simulink model "mech_airbag_vr"  (Simulink 6.0)
settings: Solver=ode45  StartTime=0.0  StopTime=3.5  RelTol=1e-6  AbsTol=1e-6
libraries: mblibv1 x38, vrlib x7, simulink x3, simulink_extras x2
settings Model: Creator=jacekk  LastModifiedBy=batserve  ExtModeAutoUpdateStatusClock=off
settings DataIOCC: SaveOutput=off  SaveTime=off  SignalLoggingName=logsOut
settings OptimizationCC: BooleanDataType=off
settings DebuggingCC: CheckExecutionContextPreStartOutputMsg=on  CheckExecutionContextRuntimeOutputMsg=on  SolverPrmCheckMsg=none
settings HardwareCC: TargetUnknown=on

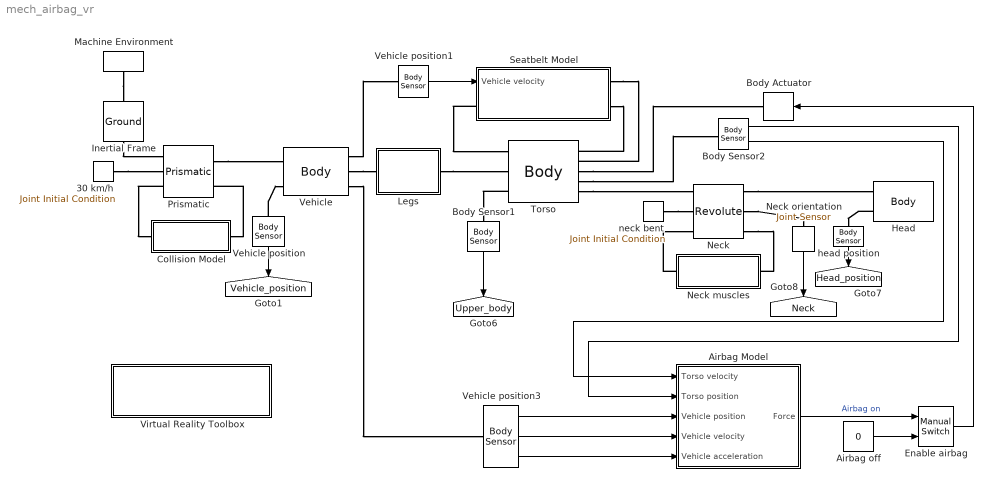
== system mech_airbag_vr ==
  30 km/h : mblibv1/Sensors &  Actuators/Joint Initial Condition  Opaque=on  PhysicalDomain=Mechanical  DialogClass=InitialConditionBlock  Primitive=P1  CoordPosition=0  Velocity=30/3.6  AngleUnits=deg  ArcVelocityUnits=deg/s  CoordPositionUnits=m  VelocityUnits=m/s  InitialConditions=P1$true$0$m$deg$30/3.6$m/s$deg/s#P2$false$0$m$rad$0$m/s$rad/s#P3$false$0$m$rad$0$m/s$rad/s#R1$false$0$m$rad$0$m/s$rad/s#R2$false$0$m$rad$0$m/s$rad/s#R3$false$0$m$rad$0$m/s$rad/s#S$false$0$m$rad$0$m/s$rad/s
  Airbag Model : Subsystem
  Airbag off : Constant  Value=0
  Body Actuator : mblibv1/Sensors &  Actuators/Body Actuator  Orientation=left  Opaque=on  PhysicalDomain=Mechanical  PortType=blob  ActuationStyle=Force  AngleUnits=deg  ArcVelocityUnits=deg/s  ArcAccelerationUnits=deg/s^2  CoordPositionUnits=m  VelocityUnits=m/s  AccelerationUnits=m/s^2  ForceUnits=N  TorqueUnits=N-m  ActiveIO=on  Width=3  DialogClass=MechanicalActuatorBlock  ReferenceFrame=Absolute (World)  Angle=off  CoordPosition=on  Force=on  Torque=off
  Body Sensor1 : mblibv1/Sensors &  Actuators/Body Sensor  Orientation=down  Opaque=on  PhysicalDomain=Mechanical  PortType=blob  Muxed=on  Pose=off  Angle=on  AngleUnits=deg  ArcVelocity=off  ArcVelocityUnits=deg/s  ArcAcceleration=off  ArcAccelerationUnits=deg/s^2  CoordPosition=on  CoordPositionUnits=cm  Velocity=off  VelocityUnits=m/s  Acceleration=off  AccelerationUnits=m/s^2  Quaternion=on  QuaternionDT=off  QuaternionDDT=off  QuaternionUnits=off  OutputVector=[ 3 ]  ActiveIO=on  Width=3  DialogClass=MechanicalSensorBlock  ReferenceFrame=Absolute (World)
  Body Sensor2 : mblibv1/Sensors &  Actuators/Body Sensor  Opaque=on  PhysicalDomain=Mechanical  PortType=blob  Muxed=off  Pose=off  Angle=on  AngleUnits=deg  ArcVelocity=off  ArcVelocityUnits=deg/s  ArcAcceleration=off  ArcAccelerationUnits=deg/s^2  CoordPosition=on  CoordPositionUnits=m  Velocity=on  VelocityUnits=m/s  Acceleration=off  AccelerationUnits=m/s^2  Quaternion=on  QuaternionDT=off  QuaternionDDT=off  QuaternionUnits=off  OutputVector=[ 3 3 ]  ActiveIO=on  Width=6  DialogClass=MechanicalSensorBlock  ReferenceFrame=Absolute (World)
  Collision Model : Subsystem
  Enable airbag : simulink/Signal Routing/Manual Switch  sw=1  action=0
  Head : mblibv1/Bodies/Body  PhysicalDomain=mechanical  SubClassName=Unknown  LeftPortType=workingframe  RightPortType=workingframe  LConnTagsString=CS1|CG  DialogClass=MechanicalBodyBlock  Mass=10  MassUnits=kg  InertiaUnits=kg*m^2  Inertia=zeros(3,3)  Shape=Cylinder  ShapeDims=[1 1]  ShapeUnits=m  ShapeUse=false  Density=1  DensityUnits=kg/m^3  DensityUse=false  CG=Left$CG$[0 15 0]$CS1$CS1$cm$[0 0 0]$Euler X-Y-Z$deg$WORLD$true  WorkingFrames=Left$CS1$[0 0 0]$ADJOINING$ADJOINING$cm$[0 0 0]$Euler X-Y-Z$deg$WORLD$true
  Inertial Frame : mblibv1/Bodies/Ground  Orientation=down  Opaque=on  LeftPortType=env  RightPortType=workingframe  PhysicalDomain=Mechanical  DialogClass=GroundBlock  CoordPosition=[0 0 0]  CoordPositionUnits=m  StateVectorMgrId=-1  MachineId=[0 0]  ShowEnvPort=on
  Legs : Subsystem
  Machine Environment : mblibv1/Bodies/Machine Environment  Tag=Factory ground  Orientation=down  DialogController=MECH.DialogSource  Opaque=on  PortType=env  PhysicalDomain=Mechanical  DialogTemplateClass=MECH.MachineEnvironment  SyncWhenCopied=off  Gravity=[0 0 0]  GravityUnits=m/s^2  GravityAsSignal=off  Dimensionality=3D Only  AnalysisType=Forward dynamics  LinearAssemblyTolerance=1e-3  LinearAssemblyToleranceUnits=m  AngularAssemblyTolerance=1e-3  AngularAssemblyToleranceUnits=rad  ConstraintSolverType=Stabilizing  ConstraintRelTolerance=1e-4  ConstraintAbsTolerance=1e-4  UseRobustSingularityHandling=off  StatePerturbationType=Adaptive  PerturbationSize=1e-3  VisualizeMachine=on
  Neck : mblibv1/Joints/Revolute  PhysicalDomain=mechanical  SubClassName=Unknown  LeftPortType=blob  RightPortType=blob  LConnTagsString=__newl0|SA1|SA2  RConnTagsString=__newr0|SA1|SA2  NumSAPorts=4  CutJoint=off  MarkAsCut=off  Primitives=revolute  PrimitiveProps=R1$Base$[0 0 1]$revolute  DialogClass=JointBlock
  Neck orientation : mblibv1/Sensors &  Actuators/Joint Sensor  Orientation=down  Opaque=on  PhysicalDomain=Mechanical  PortType=blob  Muxed=on  Pose=off  Angle=on  AngleUnits=rad  ArcVelocity=off  ArcVelocityUnits=deg/s  ArcAcceleration=off  ArcAccelerationUnits=deg/s^2  CoordPosition=on  CoordPositionUnits=m  Velocity=off  VelocityUnits=m/s  Acceleration=off  AccelerationUnits=m/s^2  Quaternion=on  QuaternionDT=off  QuaternionDDT=off  QuaternionUnits=off  OutputVector=[ 1 ]  ActiveIO=on  Width=1  DialogClass=MechanicalSensorBlock  Primitive=R1  Force=off  ForceUnits=N  Torque=off  TorqueUnits=N-m  ReferenceFrame=Absolute (INERTIAL)  ReactionSensedSide=Base  ReactionReferenceFrame=Absolute (World)  ReactionForce=off  ReactionForceUnits=N  ReactionMoment=off  ReactionMomentUnits=N-m
  Neck muscles : Subsystem  Orientation=left
  Prismatic : mblibv1/Joints/Prismatic  PhysicalDomain=mechanical  SubClassName=Unknown  LeftPortType=blob  RightPortType=blob  LConnTagsString=__newl0|SA1|SA2  RConnTagsString=__newr0|SA1  NumSAPorts=3  CutJoint=off  MarkAsCut=off  Primitives=prismatic  PrimitiveProps=P1$WORLD$[1 0 0]$prismatic  DialogClass=JointBlock
  Seatbelt Model : Subsystem
  Torso : mblibv1/Bodies/Body  PhysicalDomain=mechanical  SubClassName=Unknown  LeftPortType=workingframe  RightPortType=workingframe  LConnTagsString=CS4|CS1|CG  RConnTagsString=CS6|CS5|CS8|CS3|CS2  DialogClass=MechanicalBodyBlock  Mass=30  MassUnits=kg  InertiaUnits=kg*m^2  Inertia=zeros(3,3)  Shape=Cylinder  ShapeDims=[1 1]  ShapeUnits=m  ShapeUse=false  Density=1  DensityUnits=kg/m^3  DensityUse=false  CG=Left$CG$[0 117.5 0]$CS1$CS1$cm$[0 0 0]$Euler X-Y-Z$deg$WORLD$true  WorkingFrames=Right$CS6$[0 180 0]$CS1$CS1$cm$[0 0 0]$Euler X-Y-Z$deg$WORLD$true#Right$CS5$[0 0 0]$CS1$CS1$cm$[0 0 0]$Euler X-Y-Z$deg$WORLD$true#Left$CS4$[0 0 0]$CS1$CS1$cm$[0 0 0]$Euler X-Y-Z$deg$WORLD$true#Left$CS1$[0 0 0]$ADJOINING$ADJOINING$cm$[0 0 0]$Euler X-Y-Z$deg$WORLD$true#Right$CS8$[0 237 0]$CS1$CS1$cm$[0 0 0]$Euler X-Y-Z$deg$WORLD$true#Right$CS3$[0 237 0]$CS1$CS1$cm$[0 0 0]$Euler X-Y-Z$deg$WORLD$true#Right$CS2$[0 237 0]$CS1$CS1$cm$[0 0 0]$Euler X-Y-Z$deg$CS1$true
  Vehicle : mblibv1/Bodies/Body  PhysicalDomain=mechanical  SubClassName=Unknown  LeftPortType=workingframe  RightPortType=workingframe  LConnTagsString=CS1|CG  RConnTagsString=CS4|CS2|CS3  DialogClass=MechanicalBodyBlock  Mass=2000  MassUnits=kg  InertiaUnits=kg*m^2  Inertia=zeros(3,3)  Shape=Cylinder  ShapeDims=[1 1]  ShapeUnits=m  ShapeUse=false  Density=1  DensityUnits=kg/m^3  DensityUse=false  CG=Left$CG$[0 0 0]$WORLD$WORLD$cm$[0 0 0]$Euler X-Y-Z$deg$WORLD$true  WorkingFrames=Right$CS4$[0 0 0]$CG$CG$cm$[0 0 0]$Euler X-Y-Z$deg$WORLD$true#Left$CS1$[0 0 0]$CG$CG$cm$[0 0 0]$Euler X-Y-Z$deg$WORLD$true#Right$CS2$[10.75 -152 0]$CG$CG$cm$[0 0 0]$Euler X-Y-Z$deg$WORLD$true#Right$CS3$[0 0 0]$CG$CG$cm$[0 0 0]$Euler X-Y-Z$deg$WORLD$true
  Vehicle position : mblibv1/Sensors &  Actuators/Body Sensor  Orientation=down  Opaque=on  PhysicalDomain=Mechanical  PortType=blob  Muxed=off  Pose=off  Angle=on  AngleUnits=deg  ArcVelocity=off  ArcVelocityUnits=deg/s  ArcAcceleration=off  ArcAccelerationUnits=deg/s^2  CoordPosition=on  CoordPositionUnits=cm  Velocity=off  VelocityUnits=m/s  Acceleration=off  AccelerationUnits=m/s^2  Quaternion=on  QuaternionDT=off  QuaternionDDT=off  QuaternionUnits=off  OutputVector=[ 3 ]  ActiveIO=on  Width=3  DialogClass=MechanicalSensorBlock  ReferenceFrame=Absolute (World)
  Vehicle position1 : mblibv1/Sensors &  Actuators/Body Sensor  Opaque=on  PhysicalDomain=Mechanical  PortType=blob  Muxed=off  Pose=off  Angle=on  AngleUnits=deg  ArcVelocity=off  ArcVelocityUnits=deg/s  ArcAcceleration=off  ArcAccelerationUnits=deg/s^2  CoordPosition=off  CoordPositionUnits=cm  Velocity=on  VelocityUnits=m/s  Acceleration=off  AccelerationUnits=m/s^2  Quaternion=on  QuaternionDT=off  QuaternionDDT=off  QuaternionUnits=off  OutputVector=[ 3 ]  ActiveIO=on  Width=3  DialogClass=MechanicalSensorBlock  ReferenceFrame=Absolute (World)
  Vehicle position3 : mblibv1/Sensors &  Actuators/Body Sensor  Opaque=on  PhysicalDomain=Mechanical  PortType=blob  Muxed=off  Pose=off  Angle=on  AngleUnits=deg  ArcVelocity=off  ArcVelocityUnits=deg/s  ArcAcceleration=off  ArcAccelerationUnits=deg/s^2  CoordPosition=on  CoordPositionUnits=m  Velocity=on  VelocityUnits=m/s  Acceleration=on  AccelerationUnits=m/s^2  Quaternion=on  QuaternionDT=off  QuaternionDDT=off  QuaternionUnits=off  OutputVector=[ 3 3 3 ]  ActiveIO=on  Width=9  DialogClass=MechanicalSensorBlock  ReferenceFrame=Absolute (World)
  Virtual Reality Toolbox : Subsystem
      settings: OpenFcn=open_system([gcb '/VR Sink1']);
      mask Display: disp(sprintf('Double-click to view scene'))
  head position : mblibv1/Sensors &  Actuators/Body Sensor  Orientation=down  Opaque=on  PhysicalDomain=Mechanical  PortType=blob  Muxed=on  Pose=off  Angle=on  AngleUnits=deg  ArcVelocity=off  ArcVelocityUnits=deg/s  ArcAcceleration=off  ArcAccelerationUnits=deg/s^2  CoordPosition=on  CoordPositionUnits=cm  Velocity=off  VelocityUnits=m/s  Acceleration=off  AccelerationUnits=m/s^2  Quaternion=on  QuaternionDT=off  QuaternionDDT=off  QuaternionUnits=off  OutputVector=[ 3 ]  ActiveIO=on  Width=3  DialogClass=MechanicalSensorBlock  ReferenceFrame=Absolute (World)
  neck bent : mblibv1/Sensors &  Actuators/Joint Initial Condition  Opaque=on  PhysicalDomain=Mechanical  DialogClass=InitialConditionBlock  Primitive=R1  CoordPosition=-0.2  Velocity=0  AngleUnits=rad  ArcVelocityUnits=deg/s  CoordPositionUnits=m  VelocityUnits=m/s  InitialConditions=P1$false$0$m$rad$0$m/s$rad/s#P2$false$0$m$rad$0$m/s$rad/s#P3$false$0$m$rad$0$m/s$rad/s#R1$true$-0.2$m$rad$0$m/s$deg/s#R2$false$0$m$rad$0$m/s$rad/s#R3$false$0$m$rad$0$m/s$rad/s#S$false$0$m$rad$0$m/s$rad/s
  tag scope: Head_position=global, Neck=global, Upper_body=global, Vehicle_position=global
  wires:
  Vehicle position/1 -> [Vehicle_position]
  Body Sensor1/1 -> [Upper_body]
  head position/1 -> [Head_position]
  Neck orientation/1 -> [Neck]
  Vehicle position1/1 -> Seatbelt Model/1(Vehicle velocity)
  Vehicle position3/1 -> Airbag Model/3(Vehicle position)
  Vehicle position3/2 -> Airbag Model/4(Vehicle velocity)
  Vehicle position3/3 -> Airbag Model/5(Vehicle acceleration)
  Body Sensor2/2 -> Airbag Model/1(Torso velocity)
  Body Sensor2/1 -> Airbag Model/2(Torso position)
  Airbag Model/1(Force) -> Enable airbag/1  "Airbag on"
  Airbag off/1 -> Enable airbag/2
  Enable airbag/1 -> Body Actuator/1
  connections:
  Torso/RConn5 -- Neck/LConn1
  Neck/RConn1 -- Head/LConn1
  Inertial Frame/RConn1 -- Prismatic/LConn1
  Prismatic/RConn1 -- Vehicle/LConn1
  30 km/h/RConn1 -- Prismatic/LConn2
  Collision Model/RConn1 -- Prismatic/RConn2
  Torso/LConn3 -- Body Sensor1/LConn1
  Head/LConn2 -- head position/LConn1
  Vehicle position/LConn1 -- Vehicle/LConn2
  Neck/RConn3 -- Neck muscles/LConn1
  Neck muscles/RConn1 -- Neck/LConn3
  neck bent/RConn1 -- Neck/LConn2
  Neck/RConn2 -- Neck orientation/LConn1
  Seatbelt Model/RConn1 -- Torso/RConn2
  Vehicle/RConn1 -- Vehicle position1/LConn1
  Seatbelt Model/RConn2 -- Torso/RConn1
  Vehicle/RConn3 -- Vehicle position3/LConn1
  Prismatic/LConn3 -- Collision Model/LConn1
  Vehicle/RConn2 -- Legs/LConn1
  Seatbelt Model/LConn1 -- Torso/LConn1
  Torso/RConn4 -- Body Sensor2/LConn1
  Torso/RConn3 -- Body Actuator/RConn1
  Legs/RConn1 -- Torso/LConn2
  Machine Environment/RConn1 -- Inertial Frame/LConn1

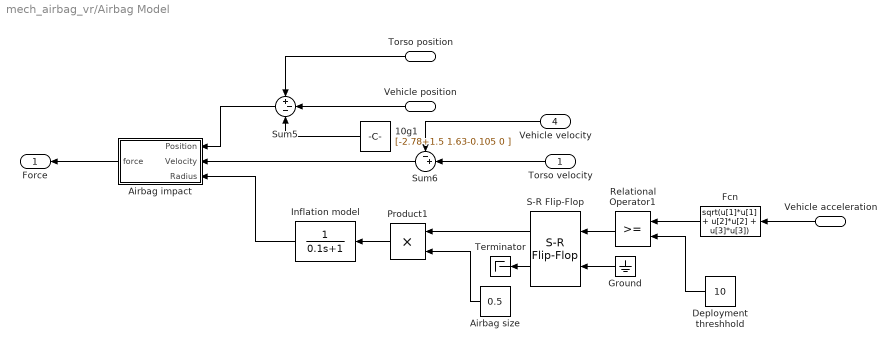
== system mech_airbag_vr/Airbag Model ==
  Torso velocity : Inport  Orientation=left  Port=1  LatchInput=off
  Torso position : Inport  Orientation=left  Port=2  LatchInput=off
  Vehicle position : Inport  Orientation=left  Port=3  LatchInput=off
  Vehicle velocity : Inport  Orientation=left  Port=4  LatchInput=off
  Vehicle acceleration : Inport  Orientation=left  Port=5  LatchInput=off
  10g1 : Constant  Orientation=left  Value=[-2.78+1.5 1.63-0.105 0 ]
  Airbag size : Constant  Orientation=left  Value=0.5
  Airbag impact : Subsystem  Orientation=left
  Deployment threshhold : Constant  Orientation=left  Value=10
  Fcn : Fcn  Orientation=left  Expr=sqrt(u[1]*u[1] + u[2]*u[2] + u[3]*u[3])
  Ground : Ground  Orientation=left
  Inflation model : TransferFcn  Orientation=left  Denominator=[0.1 1]
  Product1 : Product  Orientation=left  SaturateOnIntegerOverflow=on  InputSameDT=on
  Relational Operator1 : RelationalOperator  Orientation=left  ZeroCross=off  InputSameDT=on
  S-R Flip-Flop : simulink_extras/Flip Flops/S-R Flip-Flop  Orientation=left  initial_condition=0
  Sum5 : Sum  Orientation=left  Inputs=+--  SaturateOnIntegerOverflow=on  InputSameDT=on
  Sum6 : Sum  Orientation=left  Inputs=-+|  SaturateOnIntegerOverflow=on  InputSameDT=on
  Terminator : Terminator
  Force : Outport  Orientation=left
  wires:
  10g1/1 -> Sum5/3
  Sum6/1 -> Airbag impact/2(Velocity)
  S-R Flip-Flop/1 -> Product1/1
  Product1/1 -> Inflation model/1
  Vehicle position/1 -> Sum5/2
  Airbag impact/1(force) -> Force/1
  Relational Operator1/1 -> S-R Flip-Flop/1
  Fcn/1 -> Relational Operator1/1
  Vehicle acceleration/1 -> Fcn/1
  Torso velocity/1 -> Sum6/2
  Sum5/1 -> Airbag impact/1(Position)
  Torso position/1 -> Sum5/1
  Inflation model/1 -> Airbag impact/3(Radius)
  Airbag size/1 -> Product1/2
  Deployment threshhold/1 -> Relational Operator1/2
  Vehicle velocity/1 -> Sum6/1
  S-R Flip-Flop/2 -> Terminator/1
  Ground/1 -> S-R Flip-Flop/2

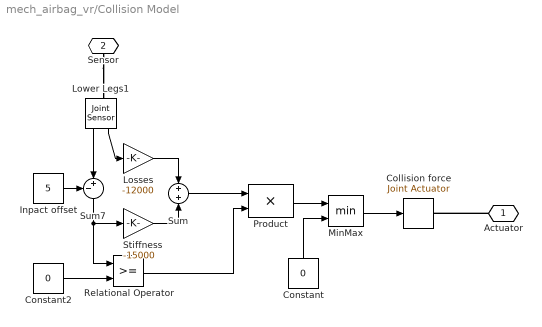
== system mech_airbag_vr/Collision Model ==
  Collision force : mblibv1/Sensors &  Actuators/Joint Actuator  Opaque=on  PhysicalDomain=Mechanical  PortType=blob  ActuationStyle=Force  AngleUnits=deg  ArcVelocityUnits=deg/s  ArcAccelerationUnits=deg/s^2  CoordPositionUnits=m  VelocityUnits=m/s  AccelerationUnits=m/s^2  ForceUnits=N  TorqueUnits=N-m  ActiveIO=on  Width=1  DialogClass=MechanicalActuatorBlock  Primitive=P1  ReferenceFrame=Absolute (INERTIAL)
  Constant : Constant  Orientation=up  Value=0
  Constant2 : Constant  Value=0
  Inpact offset : Constant  Value=5
  Losses : Gain  Gain=-12000  SaturateOnIntegerOverflow=on
  Lower Legs1 : mblibv1/Sensors &  Actuators/Joint Sensor  Orientation=down  Opaque=on  PhysicalDomain=Mechanical  PortType=blob  Muxed=off  Pose=off  Angle=on  AngleUnits=rad  ArcVelocity=off  ArcVelocityUnits=deg/s  ArcAcceleration=off  ArcAccelerationUnits=deg/s^2  CoordPosition=on  CoordPositionUnits=m  Velocity=on  VelocityUnits=m/s  Acceleration=off  AccelerationUnits=m/s^2  Quaternion=on  QuaternionDT=off  QuaternionDDT=off  QuaternionUnits=off  OutputVector=[ 1 1 ]  ActiveIO=on  Width=2  DialogClass=MechanicalSensorBlock  Primitive=P1  Force=off  ForceUnits=N  Torque=off  TorqueUnits=N-m  ReferenceFrame=Absolute (INERTIAL)  ReactionSensedSide=Base  ReactionReferenceFrame=Absolute (World)  ReactionForce=off  ReactionForceUnits=N  ReactionMoment=off  ReactionMomentUnits=N-m
  MinMax : MinMax  Inputs=2  ZeroCross=off  SaturateOnIntegerOverflow=on  InputSameDT=on
  Product : Product  SaturateOnIntegerOverflow=on  InputSameDT=on
  Relational Operator : RelationalOperator  ZeroCross=off  InputSameDT=on
  Stiffness : Gain  Gain=-15000  SaturateOnIntegerOverflow=on
  Sum : Sum  SaturateOnIntegerOverflow=on  InputSameDT=on
  Sum7 : Sum  Orientation=down  Inputs=-+|  SaturateOnIntegerOverflow=on  InputSameDT=on
  Actuator : PMIOPort  Orientation=left  Port=1  Side=Right
  Sensor : PMIOPort  Orientation=down  Port=2  Side=Left
  wires:
  MinMax/1 -> Collision force/1
  Lower Legs1/2 -> Losses/1
  Stiffness/1 -> Sum/2
  Relational Operator/1 -> Product/2
  Sum/1 -> Product/1
  Lower Legs1/1 -> Sum7/2
  Inpact offset/1 -> Sum7/1
  Sum7/1 -> Relational Operator/1, Stiffness/1
  Constant2/1 -> Relational Operator/2
  Product/1 -> MinMax/1
  Losses/1 -> Sum/1
  Constant/1 -> MinMax/2
  connections:
  Actuator/RConn1 -- Collision force/RConn1
  Sensor/RConn1 -- Lower Legs1/LConn1

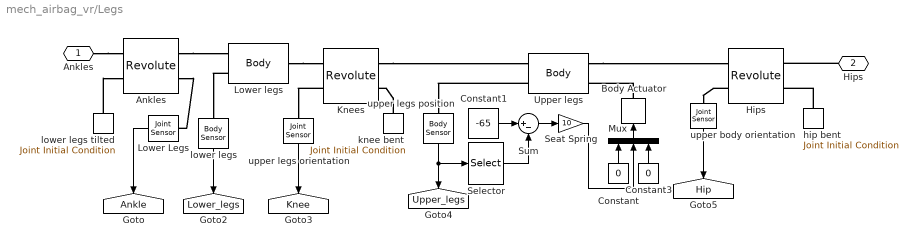
== system mech_airbag_vr/Legs ==
  Ankles : mblibv1/Joints/Revolute  PhysicalDomain=mechanical  SubClassName=Unknown  LeftPortType=blob  RightPortType=blob  LConnTagsString=__newl0|SA1  RConnTagsString=__newr0|SA1  NumSAPorts=2  CutJoint=off  MarkAsCut=off  Primitives=revolute  PrimitiveProps=R1$Base$[0 0 1]$revolute  DialogClass=JointBlock
  Body Actuator : mblibv1/Sensors &  Actuators/Body Actuator  Orientation=up  Opaque=on  PhysicalDomain=Mechanical  PortType=blob  ActuationStyle=Force  AngleUnits=deg  ArcVelocityUnits=deg/s  ArcAccelerationUnits=deg/s^2  CoordPositionUnits=m  VelocityUnits=m/s  AccelerationUnits=m/s^2  ForceUnits=N  TorqueUnits=N-m  ActiveIO=on  Width=3  DialogClass=MechanicalActuatorBlock  ReferenceFrame=Absolute (World)  Angle=off  CoordPosition=on  Force=on  Torque=off
  Constant : Constant  Orientation=up  Value=0
  Constant1 : Constant  Value=-65
  Constant3 : Constant  Orientation=up  Value=0
  Hips : mblibv1/Joints/Revolute  PhysicalDomain=mechanical  SubClassName=Unknown  LeftPortType=blob  RightPortType=blob  LConnTagsString=__newl0|SA1  RConnTagsString=__newr0|SA1  NumSAPorts=2  CutJoint=off  MarkAsCut=off  Primitives=revolute  PrimitiveProps=R1$Base$[0 0 1]$revolute  DialogClass=JointBlock
  Knees : mblibv1/Joints/Revolute  PhysicalDomain=mechanical  SubClassName=Unknown  LeftPortType=blob  RightPortType=blob  LConnTagsString=__newl0|SA1  RConnTagsString=__newr0|SA1  NumSAPorts=2  CutJoint=off  MarkAsCut=off  Primitives=revolute  PrimitiveProps=R1$Base$[0 0 1]$revolute  DialogClass=JointBlock
  Lower Legs : mblibv1/Sensors &  Actuators/Joint Sensor  Orientation=left  Opaque=on  PhysicalDomain=Mechanical  PortType=blob  Muxed=on  Pose=off  Angle=on  AngleUnits=rad  ArcVelocity=off  ArcVelocityUnits=deg/s  ArcAcceleration=off  ArcAccelerationUnits=deg/s^2  CoordPosition=on  CoordPositionUnits=m  Velocity=off  VelocityUnits=m/s  Acceleration=off  AccelerationUnits=m/s^2  Quaternion=on  QuaternionDT=off  QuaternionDDT=off  QuaternionUnits=off  OutputVector=[ 1 ]  ActiveIO=on  Width=1  DialogClass=MechanicalSensorBlock  Primitive=R1  Force=off  ForceUnits=N  Torque=off  TorqueUnits=N-m  ReferenceFrame=Absolute (INERTIAL)  ReactionSensedSide=Base  ReactionReferenceFrame=Absolute (World)  ReactionForce=off  ReactionForceUnits=N  ReactionMoment=off  ReactionMomentUnits=N-m
  Lower legs : mblibv1/Bodies/Body  PhysicalDomain=mechanical  SubClassName=Unknown  LeftPortType=workingframe  RightPortType=workingframe  LConnTagsString=CS1|CG  RConnTagsString=CS2  DialogClass=MechanicalBodyBlock  Mass=5  MassUnits=kg  InertiaUnits=kg*m^2  Inertia=zeros(3,3)  Shape=Cylinder  ShapeDims=[1 1]  ShapeUnits=m  ShapeUse=false  Density=1  DensityUnits=kg/m^3  DensityUse=false  CG=Left$CG$[0 60 0]$CS1$CS1$cm$[0 0 0]$Euler X-Y-Z$deg$CS1$true  WorkingFrames=Left$CS1$[0 0 0]$ADJOINING$ADJOINING$cm$[0 0 0]$Euler X-Y-Z$deg$ADJOINING$true#Right$CS2$[0 120 0]$CS1$CS1$cm$[0 0 0]$Euler X-Y-Z$deg$CS1$true
  Mux : Mux  Orientation=up  Inputs=3
  Seat Spring : Gain  Gain=10  SaturateOnIntegerOverflow=on
  Selector : Selector  Elements=2  InputPortWidth=3
  Sum : Sum  Inputs=|+-  SaturateOnIntegerOverflow=on  InputSameDT=on
  Upper legs : mblibv1/Bodies/Body  PhysicalDomain=mechanical  SubClassName=Unknown  LeftPortType=workingframe  RightPortType=workingframe  LConnTagsString=CS1|CG  RConnTagsString=CS2|CS3  DialogClass=MechanicalBodyBlock  Mass=15  MassUnits=kg  InertiaUnits=kg*m^2  Inertia=zeros(3,3)  Shape=Cylinder  ShapeDims=[1 1]  ShapeUnits=m  ShapeUse=false  Density=1  DensityUnits=kg/m^3  DensityUse=false  CG=Left$CG$[0 94 0]$CS1$CS1$cm$[0 0 0]$Euler X-Y-Z$deg$CS1$true  WorkingFrames=Left$CS1$[0 0 0]$ADJOINING$ADJOINING$cm$[0 0 0]$Euler X-Y-Z$deg$ADJOINING$true#Right$CS2$[0 188 0]$CS1$CS1$cm$[0 0 0]$Euler X-Y-Z$deg$CS1$true#Right$CS3$[0 188 0]$CS1$CS1$cm$[0 0 0]$Euler X-Y-Z$deg$CS1$true
  hip bent : mblibv1/Sensors &  Actuators/Joint Initial Condition  Orientation=up  Opaque=on  PhysicalDomain=Mechanical  DialogClass=InitialConditionBlock  Primitive=R1  CoordPosition=-1.57  Velocity=0  AngleUnits=rad  ArcVelocityUnits=deg/s  CoordPositionUnits=m  VelocityUnits=m/s  InitialConditions=P1$false$0$m$rad$0$m/s$rad/s#P2$false$0$m$rad$0$m/s$rad/s#P3$false$0$m$rad$0$m/s$rad/s#R1$true$-1.57$m$rad$0$m/s$deg/s#R2$false$0$m$rad$0$m/s$rad/s#R3$false$0$m$rad$0$m/s$rad/s#S$false$0$m$rad$0$m/s$rad/s
  knee bent : mblibv1/Sensors &  Actuators/Joint Initial Condition  Orientation=up  Opaque=on  PhysicalDomain=Mechanical  DialogClass=InitialConditionBlock  Primitive=R1  CoordPosition=1.27  Velocity=0  AngleUnits=rad  ArcVelocityUnits=deg/s  CoordPositionUnits=m  VelocityUnits=m/s  InitialConditions=P1$false$0$m$rad$0$m/s$rad/s#P2$false$0$m$rad$0$m/s$rad/s#P3$false$0$m$rad$0$m/s$rad/s#R1$true$1.27$m$rad$0$m/s$deg/s#R2$false$0$m$rad$0$m/s$rad/s#R3$false$0$m$rad$0$m/s$rad/s#S$false$0$m$rad$0$m/s$rad/s
  "lower legs " : mblibv1/Sensors &  Actuators/Body Sensor  Orientation=down  Opaque=on  PhysicalDomain=Mechanical  PortType=blob  Muxed=on  Pose=off  Angle=on  AngleUnits=deg  ArcVelocity=off  ArcVelocityUnits=deg/s  ArcAcceleration=off  ArcAccelerationUnits=deg/s^2  CoordPosition=on  CoordPositionUnits=cm  Velocity=off  VelocityUnits=m/s  Acceleration=off  AccelerationUnits=m/s^2  Quaternion=on  QuaternionDT=off  QuaternionDDT=off  QuaternionUnits=off  OutputVector=[ 3 ]  ActiveIO=on  Width=3  DialogClass=MechanicalSensorBlock  ReferenceFrame=Absolute (World)
  lower legs tilted : mblibv1/Sensors &  Actuators/Joint Initial Condition  Orientation=up  Opaque=on  PhysicalDomain=Mechanical  DialogClass=InitialConditionBlock  Primitive=R1  CoordPosition=0.5  Velocity=0  AngleUnits=rad  ArcVelocityUnits=deg/s  CoordPositionUnits=m  VelocityUnits=m/s  InitialConditions=P1$false$0$m$rad$0$m/s$rad/s#P2$false$0$m$rad$0$m/s$rad/s#P3$false$0$m$rad$0$m/s$rad/s#R1$true$0.5$m$rad$0$m/s$deg/s#R2$false$0$m$rad$0$m/s$rad/s#R3$false$0$m$rad$0$m/s$rad/s#S$false$0$m$rad$0$m/s$rad/s
  upper body orientation : mblibv1/Sensors &  Actuators/Joint Sensor  Orientation=down  Opaque=on  PhysicalDomain=Mechanical  PortType=blob  Muxed=on  Pose=off  Angle=on  AngleUnits=rad  ArcVelocity=off  ArcVelocityUnits=deg/s  ArcAcceleration=off  ArcAccelerationUnits=deg/s^2  CoordPosition=on  CoordPositionUnits=m  Velocity=off  VelocityUnits=m/s  Acceleration=off  AccelerationUnits=m/s^2  Quaternion=on  QuaternionDT=off  QuaternionDDT=off  QuaternionUnits=off  OutputVector=[ 1 ]  ActiveIO=on  Width=1  DialogClass=MechanicalSensorBlock  Primitive=R1  Force=off  ForceUnits=N  Torque=off  TorqueUnits=N-m  ReferenceFrame=Absolute (INERTIAL)  ReactionSensedSide=Base  ReactionReferenceFrame=Absolute (World)  ReactionForce=off  ReactionForceUnits=N  ReactionMoment=off  ReactionMomentUnits=N-m
  upper legs orientation : mblibv1/Sensors &  Actuators/Joint Sensor  Orientation=down  Opaque=on  PhysicalDomain=Mechanical  PortType=blob  Muxed=on  Pose=off  Angle=on  AngleUnits=rad  ArcVelocity=off  ArcVelocityUnits=deg/s  ArcAcceleration=off  ArcAccelerationUnits=deg/s^2  CoordPosition=on  CoordPositionUnits=m  Velocity=off  VelocityUnits=m/s  Acceleration=off  AccelerationUnits=m/s^2  Quaternion=on  QuaternionDT=off  QuaternionDDT=off  QuaternionUnits=off  OutputVector=[ 1 ]  ActiveIO=on  Width=1  DialogClass=MechanicalSensorBlock  Primitive=R1  Force=off  ForceUnits=N  Torque=off  TorqueUnits=N-m  ReferenceFrame=Absolute (INERTIAL)  ReactionSensedSide=Base  ReactionReferenceFrame=Absolute (World)  ReactionForce=off  ReactionForceUnits=N  ReactionMoment=off  ReactionMomentUnits=N-m
  upper legs position : mblibv1/Sensors &  Actuators/Body Sensor  Orientation=down  Opaque=on  PhysicalDomain=Mechanical  PortType=blob  Muxed=on  Pose=off  Angle=on  AngleUnits=deg  ArcVelocity=off  ArcVelocityUnits=deg/s  ArcAcceleration=off  ArcAccelerationUnits=deg/s^2  CoordPosition=on  CoordPositionUnits=cm  Velocity=off  VelocityUnits=m/s  Acceleration=off  AccelerationUnits=m/s^2  Quaternion=on  QuaternionDT=off  QuaternionDDT=off  QuaternionUnits=off  OutputVector=[ 3 ]  ActiveIO=on  Width=3  DialogClass=MechanicalSensorBlock  ReferenceFrame=Absolute (World)
  "Ankles  " : PMIOPort  Port=1  Side=Left
  "Hips " : PMIOPort  Orientation=left  Port=2  Side=Right
  tag scope: Ankle=global, Hip=global, Knee=global, Lower_legs=global, Upper_legs=global
  wires:
  Lower Legs/1 -> [Ankle]
  "lower legs "/1 -> [Lower_legs]
  upper legs orientation/1 -> [Knee]
  upper legs position/1 -> [Upper_legs], Selector/1
  upper body orientation/1 -> [Hip]
  Constant1/1 -> Sum/1
  Selector/1 -> Sum/2
  Sum/1 -> Seat Spring/1
  Mux/1 -> Body Actuator/1
  Constant/1 -> Mux/1
  Constant3/1 -> Mux/3
  Seat Spring/1 -> Mux/2
  connections:
  Lower legs/RConn1 -- Knees/LConn1
  Knees/RConn1 -- Upper legs/LConn1
  Upper legs/RConn1 -- Hips/LConn1
  knee bent/RConn1 -- Knees/RConn2
  hip bent/RConn1 -- Hips/RConn2
  Lower legs/LConn2 -- "lower legs "/LConn1
  Upper legs/LConn2 -- upper legs position/LConn1
  Hips/LConn2 -- upper body orientation/LConn1
  Ankles/RConn1 -- Lower legs/LConn1
  lower legs tilted/RConn1 -- Ankles/LConn2
  Ankles/RConn2 -- Lower Legs/LConn1
  Knees/LConn2 -- upper legs orientation/LConn1
  "Ankles  "/RConn1 -- Ankles/LConn1
  "Hips "/RConn1 -- Hips/RConn1
  Body Actuator/RConn1 -- Upper legs/RConn2

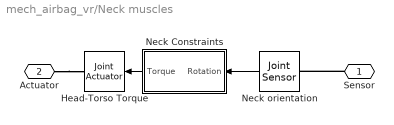
== system mech_airbag_vr/Neck muscles ==
  Head-Torso Torque : mblibv1/Sensors &  Actuators/Joint Actuator  Orientation=left  Opaque=on  PhysicalDomain=Mechanical  PortType=blob  ActuationStyle=Force  AngleUnits=deg  ArcVelocityUnits=deg/s  ArcAccelerationUnits=deg/s^2  CoordPositionUnits=m  VelocityUnits=m/s  AccelerationUnits=m/s^2  ForceUnits=N  TorqueUnits=N-m  ActiveIO=on  Width=1  DialogClass=MechanicalActuatorBlock  Primitive=R1  ReferenceFrame=Absolute (INERTIAL)
  Neck Constraints : Subsystem  Orientation=left
  Neck orientation : mblibv1/Sensors &  Actuators/Joint Sensor  Orientation=left  Opaque=on  PhysicalDomain=Mechanical  PortType=blob  Muxed=on  Pose=off  Angle=on  AngleUnits=rad  ArcVelocity=on  ArcVelocityUnits=rad/s  ArcAcceleration=off  ArcAccelerationUnits=deg/s^2  CoordPosition=on  CoordPositionUnits=m  Velocity=off  VelocityUnits=m/s  Acceleration=off  AccelerationUnits=m/s^2  Quaternion=on  QuaternionDT=off  QuaternionDDT=off  QuaternionUnits=off  OutputVector=[ 1 1 ]  ActiveIO=on  Width=2  DialogClass=MechanicalSensorBlock  Primitive=R1  Force=off  ForceUnits=N  Torque=off  TorqueUnits=N-m  ReferenceFrame=Absolute (INERTIAL)  ReactionSensedSide=Base  ReactionReferenceFrame=Absolute (World)  ReactionForce=off  ReactionForceUnits=N  ReactionMoment=off  ReactionMomentUnits=N-m
  Sensor : PMIOPort  Orientation=left  Port=1  Side=Left
  Actuator : PMIOPort  Port=2  Side=Right
  wires:
  Neck Constraints/1(Torque) -> Head-Torso Torque/1
  Neck orientation/1 -> Neck Constraints/1(Rotation)
  connections:
  Sensor/RConn1 -- Neck orientation/LConn1
  Actuator/RConn1 -- Head-Torso Torque/RConn1

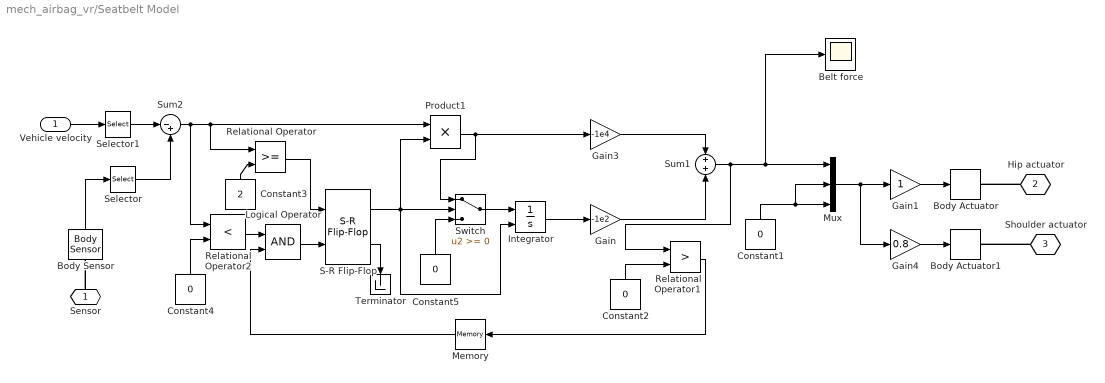
== system mech_airbag_vr/Seatbelt Model ==
  Vehicle velocity : Inport  Port=1  LatchInput=off
  Belt force : Scope
      settings: TimeRange=1  YMin=-25000  YMax=5000
  Body Actuator : mblibv1/Sensors &  Actuators/Body Actuator  Opaque=on  PhysicalDomain=Mechanical  PortType=blob  ActuationStyle=Force  AngleUnits=deg  ArcVelocityUnits=deg/s  ArcAccelerationUnits=deg/s^2  CoordPositionUnits=m  VelocityUnits=m/s  AccelerationUnits=m/s^2  ForceUnits=N  TorqueUnits=N-m  ActiveIO=on  Width=3  DialogClass=MechanicalActuatorBlock  ReferenceFrame=Local (Body CS)  Angle=off  CoordPosition=on  Force=on  Torque=off
  Body Actuator1 : mblibv1/Sensors &  Actuators/Body Actuator  Opaque=on  PhysicalDomain=Mechanical  PortType=blob  ActuationStyle=Force  AngleUnits=deg  ArcVelocityUnits=deg/s  ArcAccelerationUnits=deg/s^2  CoordPositionUnits=m  VelocityUnits=m/s  AccelerationUnits=m/s^2  ForceUnits=N  TorqueUnits=N-m  ActiveIO=on  Width=3  DialogClass=MechanicalActuatorBlock  ReferenceFrame=Absolute (World)  Angle=off  CoordPosition=on  Force=on  Torque=off
  Body Sensor : mblibv1/Sensors &  Actuators/Body Sensor  Orientation=up  Opaque=on  PhysicalDomain=Mechanical  PortType=blob  Muxed=off  Pose=off  Angle=on  AngleUnits=deg  ArcVelocity=off  ArcVelocityUnits=deg/s  ArcAcceleration=off  ArcAccelerationUnits=deg/s^2  CoordPosition=off  CoordPositionUnits=cm  Velocity=on  VelocityUnits=m/s  Acceleration=off  AccelerationUnits=m/s^2  Quaternion=on  QuaternionDT=off  QuaternionDDT=off  QuaternionUnits=off  OutputVector=[ 3 ]  ActiveIO=on  Width=3  DialogClass=MechanicalSensorBlock  ReferenceFrame=Absolute (World)
  Constant{1..2,4..5} (4 alike) : Constant  Orientation=up  Value=0
  Constant3 : Constant  Orientation=up  Value=2
  Gain : Gain  Gain=-1e2  SaturateOnIntegerOverflow=on
  Gain1 : Gain  SaturateOnIntegerOverflow=on
  Gain3 : Gain  Gain=-1e4  SaturateOnIntegerOverflow=on
  Gain4 : Gain  Gain=0.8  SaturateOnIntegerOverflow=on
  Integrator : Integrator  ExternalReset=either  AbsoluteTolerance=1e-8  ZeroCross=off
  Logical Operator : Logic
  Memory : Memory  Orientation=left
  Mux : Mux  Inputs=3
  Product1 : Product  SaturateOnIntegerOverflow=on  InputSameDT=on
  Relational Operator : RelationalOperator  ZeroCross=off  InputSameDT=on
  Relational Operator1 : RelationalOperator  Operator=>  ZeroCross=off  InputSameDT=on
  Relational Operator2 : RelationalOperator  Operator=<  ZeroCross=off  InputSameDT=on
  S-R Flip-Flop : simulink_extras/Flip Flops/S-R Flip-Flop  initial_condition=0
  Selector : Selector  InputPortWidth=3
  Selector1 : Selector  InputPortWidth=3
  Sum1 : Sum  SaturateOnIntegerOverflow=on  InputSameDT=on
  Sum2 : Sum  Inputs=|-+  SaturateOnIntegerOverflow=on  InputSameDT=on
  Switch : Switch  ZeroCross=off  InputSameDT=on
  Terminator : Terminator
      settings: Orientation=down
  Sensor : PMIOPort  Orientation=up  Port=1  Side=Left
  Hip actuator : PMIOPort  Orientation=left  Port=2  Side=Right
  Shoulder actuator : PMIOPort  Orientation=left  Port=3  Side=Right
  wires:
  Vehicle velocity/1 -> Selector1/1
  Gain1/1 -> Body Actuator/1
  Relational Operator/1 -> S-R Flip-Flop/1
  Constant3/1 -> Relational Operator/2
  Sum1/1 -> Relational Operator1/1, Mux/1, Belt force/1
  Constant1/1 -> Mux/3, Mux/2
  Constant2/1 -> Relational Operator1/2
  Body Sensor/1 -> Selector/1
  Integrator/1 -> Gain/1
  Gain/1 -> Sum1/2
  S-R Flip-Flop/1 -> Product1/2, Switch/2, Integrator/2
  Logical Operator/1 -> S-R Flip-Flop/2
  Relational Operator2/1 -> Logical Operator/1
  Relational Operator1/1 -> Memory/1
  Gain3/1 -> Sum1/1
  Mux/1 -> Gain1/1, Gain4/1
  Memory/1 -> Logical Operator/2
  Selector1/1 -> Sum2/1
  Selector/1 -> Sum2/2
  Sum2/1 -> Relational Operator2/1, Relational Operator/1, Product1/1
  Constant4/1 -> Relational Operator2/2
  Gain4/1 -> Body Actuator1/1
  Product1/1 -> Gain3/1, Switch/1
  Switch/1 -> Integrator/1
  Constant5/1 -> Switch/3
  S-R Flip-Flop/2 -> Terminator/1
  connections:
  Sensor/RConn1 -- Body Sensor/LConn1
  Hip actuator/RConn1 -- Body Actuator/RConn1
  Shoulder actuator/RConn1 -- Body Actuator1/RConn1

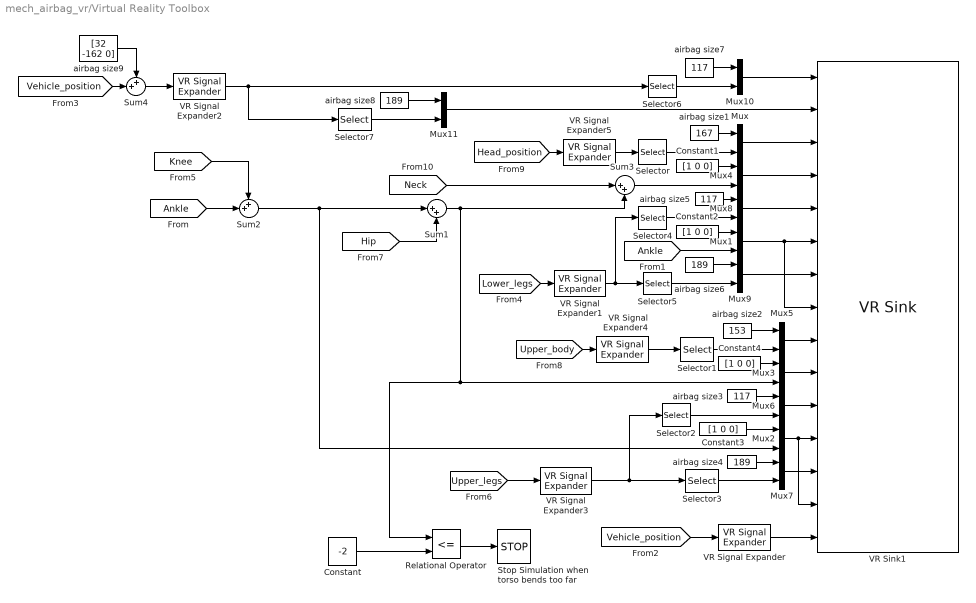
== system mech_airbag_vr/Virtual Reality Toolbox ==
  Constant : Constant  Value=-2
  Constant{1..4} (4 alike) : Constant  Value=[1 0 0]
  Mux{,1..11} (12 alike) : Mux  Inputs=2
  Relational Operator : RelationalOperator  Operator=<=  ZeroCross=off  InputSameDT=on
  Selector{,1..7} (8 alike) : Selector  Elements=[2 3]  InputPortWidth=3
  Stop Simulation when torso bends too far : Stop
  Sum1 : Sum  Inputs=|++  SaturateOnIntegerOverflow=on  InputSameDT=on
  Sum2 : Sum  Inputs=++|  SaturateOnIntegerOverflow=on  InputSameDT=on
  Sum3 : Sum  Inputs=|++  SaturateOnIntegerOverflow=on  InputSameDT=on
  Sum4 : Sum  Inputs=++|  SaturateOnIntegerOverflow=on  InputSameDT=on
  VR Signal Expander{,1..5} (6 alike) : vrlib/VR Signal Expander  outwidth=3  outidx=[2 3 1]
  VR Sink1 : vrlib/VR Sink  SampleTime=0.05  ViewEnable=on  RemoteChange=off  RemoteView=off  FieldsWritten=footL.translation#footR.translation#headCOG.translation#headROT.rotation#lowerlegL.translation#lowerlegLROT.rotation#lowerlegR.translation#lowerlegRROT.rotation#torsoCOG.translation#torsoROT.rotation#upperlegL.translation#upperlegLROT.rotation#upperlegR.translation#upperlegRROT.rotation#vehicle.translation  WorldFileName=mech_airbag_world.wrl  WorldDescription=Passenger Collision Model  AutoView=off  FigureProperties={}
  airbag size1 : Constant  Value=167
  airbag size2 : Constant  Value=153
  airbag size3 : Constant  Value=117
  airbag size4 : Constant  Value=189
  airbag size5 : Constant  Value=117
  airbag size6 : Constant  Value=189
  airbag size7 : Constant  Value=117
  airbag size8 : Constant  Value=189
  airbag size9 : Constant  Value=[32 -162 0]
  wires:
  Sum3/1 -> Mux4/2
  Mux4/1 -> VR Sink1/4
  Mux3/1 -> VR Sink1/10
  airbag size1/1 -> Mux/1
  Selector/1 -> Mux/2
  Mux/1 -> VR Sink1/3
  Selector1/1 -> Mux5/2
  airbag size3/1 -> Mux6/1
  airbag size4/1 -> Mux7/1
  airbag size6/1 -> Mux9/1
  Selector4/1 -> Mux8/2
  Selector5/1 -> Mux9/2
  Selector7/1 -> Mux11/2
  airbag size8/1 -> Mux11/1
  airbag size7/1 -> Mux10/1
  [Ankle] -> Sum2/2
  [Ankle] -> Mux1/2
  [Vehicle_position] -> VR Signal Expander/1
  [Vehicle_position] -> Sum4/2
  Sum4/1 -> VR Signal Expander2/1
  airbag size9/1 -> Sum4/1
  [Lower_legs] -> VR Signal Expander1/1
  [Hip] -> Sum1/2
  [Upper_body] -> VR Signal Expander4/1
  [Head_position] -> VR Signal Expander5/1
  [Neck] -> Sum3/1
  Selector6/1 -> Mux10/2
  VR Signal Expander2/1 -> Selector7/1, Selector6/1
  VR Signal Expander5/1 -> Selector/1
  Mux10/1 -> VR Sink1/1
  Mux11/1 -> VR Sink1/2
  Constant1/1 -> Mux4/1
  Mux8/1 -> VR Sink1/5
  airbag size5/1 -> Mux8/1
  Mux9/1 -> VR Sink1/7
  Mux1/1 -> VR Sink1/6, VR Sink1/8
  Constant2/1 -> Mux1/1
  Constant4/1 -> Mux3/1
  VR Signal Expander1/1 -> Selector5/1, Selector4/1
  Mux5/1 -> VR Sink1/9
  airbag size2/1 -> Mux5/1
  VR Signal Expander4/1 -> Selector1/1
  Constant3/1 -> Mux2/1
  Mux2/1 -> VR Sink1/12, VR Sink1/14
  [Knee] -> Sum2/1
  Sum1/1 -> Sum3/2, Relational Operator/1, Mux3/2
  Sum2/1 -> Sum1/1, Mux2/2
  Mux6/1 -> VR Sink1/11
  Selector2/1 -> Mux6/2
  Mux7/1 -> VR Sink1/13
  Selector3/1 -> Mux7/2
  VR Signal Expander/1 -> VR Sink1/15
  VR Signal Expander3/1 -> Selector3/1, Selector2/1
  [Upper_legs] -> VR Signal Expander3/1
  Constant/1 -> Relational Operator/2
  Relational Operator/1 -> Stop Simulation when torso bends too far/1

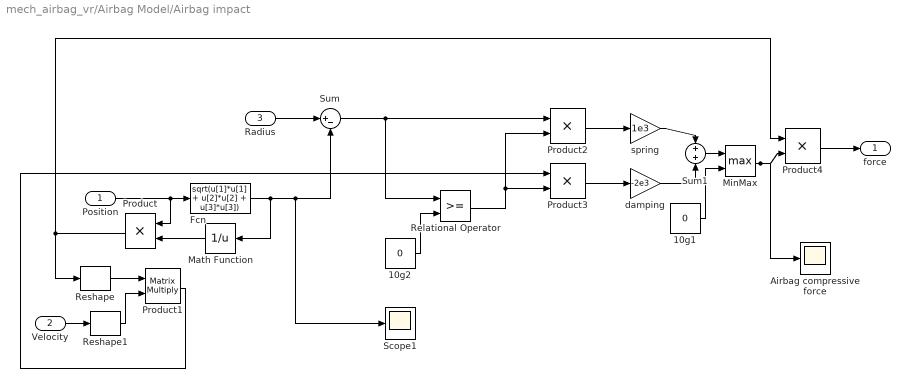
== system mech_airbag_vr/Airbag Model/Airbag impact ==
  Position : Inport  Port=1  LatchInput=off
  Velocity : Inport  Port=2  LatchInput=off
  Radius : Inport  Port=3  LatchInput=off
  10g1 : Constant  Value=0
  10g2 : Constant  Value=0
  Airbag compressive force : Scope
      settings: YMin=-1  YMax=1
  Fcn : Fcn  Expr=sqrt(u[1]*u[1] + u[2]*u[2] + u[3]*u[3])
  Math Function : Math  Orientation=left  Operator=reciprocal  SaturateOnIntegerOverflow=on
  MinMax : MinMax  Function=max  Inputs=2  ZeroCross=off  SaturateOnIntegerOverflow=on  InputSameDT=on
  Product : Product  Orientation=left  SaturateOnIntegerOverflow=on  InputSameDT=on
  Product1 : Product  Multiplication=Matrix(*)  SaturateOnIntegerOverflow=on  InputSameDT=on
  Product2 : Product  SaturateOnIntegerOverflow=on  InputSameDT=on
  Product3 : Product  SaturateOnIntegerOverflow=on  InputSameDT=on
  Product4 : Product  SaturateOnIntegerOverflow=on  InputSameDT=on
  Relational Operator : RelationalOperator  ZeroCross=off  InputSameDT=on
  Reshape : simulink/Math Operations/Reshape  OutputDimensionality=Row vector  OutputDimensions=[1,1]
  Reshape1 : simulink/Math Operations/Reshape  OutputDimensionality=Column vector  OutputDimensions=[1,1]
  Scope1 : Scope
      settings: YMin=0.25  YMax=1.75  SaveName=ScopeData4
  Sum : Sum  Inputs=|+-  SaturateOnIntegerOverflow=on  InputSameDT=on
  Sum1 : Sum  SaturateOnIntegerOverflow=on  InputSameDT=on
  damping : Gain  Gain=-2e3  SaturateOnIntegerOverflow=on
  spring : Gain  Gain=1e3  SaturateOnIntegerOverflow=on
  force : Outport
  wires:
  Position/1 -> Fcn/1, Product/1
  Fcn/1 -> Math Function/1, Sum/2, Scope1/1
  Math Function/1 -> Product/2
  Product/1 -> Reshape/1, Product4/1
  Reshape/1 -> Product1/1
  Radius/1 -> Sum/1
  10g2/1 -> Relational Operator/2
  Sum/1 -> Relational Operator/1, Product2/1
  Relational Operator/1 -> Product3/2, Product2/2
  Product2/1 -> spring/1
  Product3/1 -> damping/1
  Product1/1 -> Product3/1
  spring/1 -> Sum1/1
  damping/1 -> Sum1/2
  Product4/1 -> force/1
  Sum1/1 -> MinMax/1
  MinMax/1 -> Product4/2, Airbag compressive force/1
  10g1/1 -> MinMax/2
  Velocity/1 -> Reshape1/1
  Reshape1/1 -> Product1/2

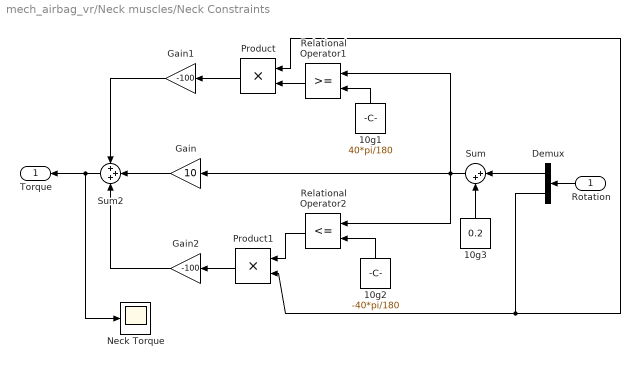
== system mech_airbag_vr/Neck muscles/Neck Constraints ==
  Rotation : Inport  Orientation=left  Port=1  LatchInput=off
  10g1 : Constant  Orientation=up  Value=40*pi/180
  10g2 : Constant  Orientation=up  Value=-40*pi/180
  10g3 : Constant  Orientation=up  Value=0.2
  Demux : Demux  Orientation=left  Outputs=2
  Gain : Gain  Orientation=left  Gain=10  SaturateOnIntegerOverflow=on
  Gain1 : Gain  Orientation=left  Gain=-100  SaturateOnIntegerOverflow=on
  Gain2 : Gain  Orientation=left  Gain=-100  SaturateOnIntegerOverflow=on
  Neck Torque : Scope
      settings: TimeRange=1  YMin=-500  YMax=2000  SaveName=ScopeData2
  Product : Product  Orientation=left  SaturateOnIntegerOverflow=on  InputSameDT=on
  Product1 : Product  Orientation=left  SaturateOnIntegerOverflow=on  InputSameDT=on
  Relational Operator1 : RelationalOperator  Orientation=left  ZeroCross=off  InputSameDT=on
  Relational Operator2 : RelationalOperator  Orientation=left  Operator=<=  ZeroCross=off  InputSameDT=on
  Sum : Sum  Orientation=left  Inputs=|++  SaturateOnIntegerOverflow=on  InputSameDT=on
  Sum2 : Sum  Orientation=left  Inputs=+++  SaturateOnIntegerOverflow=on  InputSameDT=on
  Torque : Outport  Orientation=left
  wires:
  Product/1 -> Gain1/1
  Relational Operator2/1 -> Product1/1
  Product1/1 -> Gain2/1
  Gain/1 -> Sum2/2
  Gain1/1 -> Sum2/1
  Gain2/1 -> Sum2/3
  Sum2/1 -> Torque/1, Neck Torque/1
  Rotation/1 -> Demux/1
  Relational Operator1/1 -> Product/2
  10g1/1 -> Relational Operator1/2
  10g2/1 -> Relational Operator2/2
  Demux/2 -> Product1/2, Product/1
  Demux/1 -> Sum/1
  10g3/1 -> Sum/2
  Sum/1 -> Relational Operator2/1, Gain/1, Relational Operator1/1
